simulink model "cloop_AW_1"  (Simulink 7.8)
settings: Solver=FixedStepDiscrete  StartTime=0.0  StopTime=20  FixedStep=ts  RelTol=1e-3
values from neighbouring files (symbols this model uses):
  D_aw = value(U)\value(X)    [AW_synthesis_LMI.m]    (also in Degenerator_test.m = [0 0 0 0])
  satValue = 3.6    [AW_synthesis_LMI.m]    (also in Degenerator_test.m)
  setPoint = 0.015    [Degenerator_test.m]
  ts = 0.005    [identificazione_freq.m]
undefined symbols (not defined in the file or in its folder): N2signal, satSafe
libraries: cstblocks x1
settings Model: Creator=albertoforner  LastModifiedBy=giamm  SimulationMode=external  ExtModeTrigDuration=100000  ExtModeWriteAllDataToWs=on
settings DataIOCC: LimitDataPoints=off
settings DebuggingCC: FrameProcessingCompatibilityMsg=error  StrictBusMsg=Warning
settings HardwareCC: ProdBitPerPointer=64  ProdLargestAtomicFloat=Float  ProdIntDivRoundTo=Zero  ProdEndianess=LittleEndian  ProdHWDeviceType=Specified
settings RTWCC: SystemTargetFile=rtwin.tlc  TemplateMakefile=rtwin.tmf  Description=Simulink Desktop Real-Time  RTWCompilerOptimization=On
settings CodeAppCC: MaxIdLength=95  CustomSymbolStrType=$N$R$M_T
settings RTWinTargetCC: TargetPreCompLibLocation=C:\Program Files\MATLAB\R2016b\toolbox\sldrt\lib\win64  TargetFunctionLibrary=C89/C90 (ANSI)  GeneratePreprocessorConditionals=Use local settings  UseToolchainInfoCompliant=off  ExtModeMexFile=sldrtext

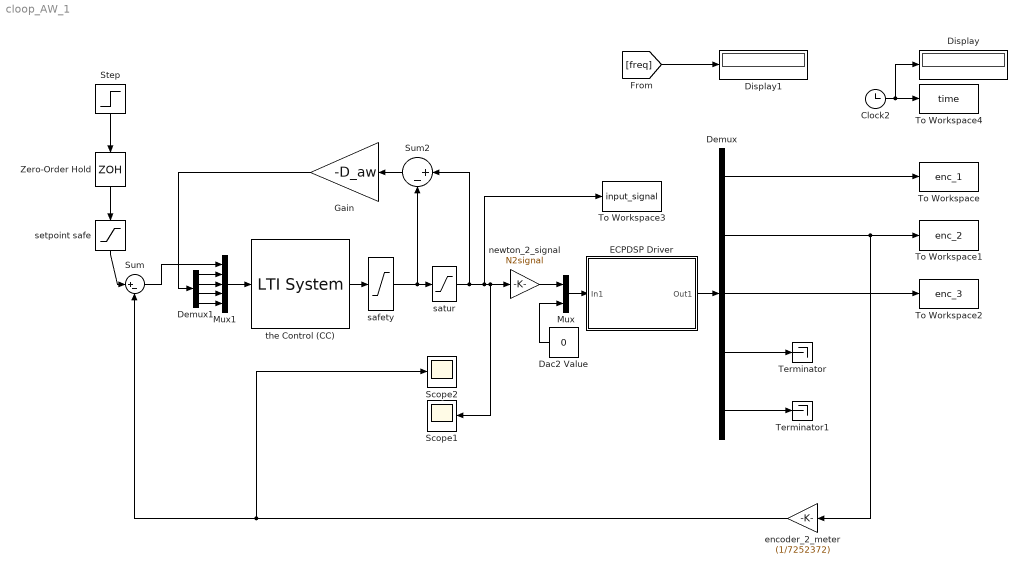
== system cloop_AW_1 ==
  Clock2 : Clock
      settings: DisableCoverage=on
  Dac2 Value : Constant  Value=0  SampleTime=ts
  Demux : Demux  Outputs=5
  Demux1 : Demux
  Display : Display
      settings: Decimation=100
  Display1 : Display
      settings: Decimation=100
  ECPDSP Driver : Subsystem  mask{BaseAddr='0xDE00', STime=ts, TimeOutPer=500, HWAccess=on}
      mask prompts: BaseAddr "Base I/O Address"; STime "Sample Time (Sec)"; TimeOutPer "Timeout Period (500 ~ 2000)"; HWAccess "Hardware Access"
      mask Display: color('black');disp('ECPDSP Driver\n upto\n 4 Encs(ADC Channels)\n and 2 Dacs')
  Gain : Gain  Gain=-D_aw
  Mux : Mux  Inputs=2
  Mux1 : Mux  Inputs=5
  Scope1 : Scope
      settings: TimeRange=auto  MaxDataPoints=5000  SaveToWorkspace=off  YMin=3.5625  YMax=3.9375  SampleTime=-1
  Scope2 : Scope
      settings: TimeRange=auto  MaxDataPoints=5000  SaveToWorkspace=off  SaveName=ScopeData  YMin=-0.03  YMax=0.0275  SampleTime=-1
  Step : Step  Time=ts  After=setPoint  SampleTime=ts
  Sum : Sum  Inputs=|+-
  Sum2 : Sum  Inputs=|+-
  Terminator : Terminator
  Terminator1 : Terminator
  To Workspace : ToWorkspace  VariableName=enc_1  SampleTime=-1
  To Workspace1 : ToWorkspace  VariableName=enc_2  SampleTime=-1
  To Workspace2 : ToWorkspace  VariableName=enc_3  SampleTime=-1
  To Workspace3 : ToWorkspace  VariableName=input_signal  SampleTime=ts
  To Workspace4 : ToWorkspace  VariableName=time  SampleTime=-1
  Zero-Order Hold : ZeroOrderHold  SampleTime=ts
  encoder_2_meter : Gain  Gain=(1/7252372)
  newton_2_signal : Gain  Gain=N2signal
  safety : Saturate  UpperLimit=satSafe  LowerLimit=-satSafe
  satur : Saturate  UpperLimit=satValue  LowerLimit=-satValue
  setpoint safe : Saturate  UpperLimit=0.02  LowerLimit=-0.02
  the Control (CC) : cstblocks/LTI System  sys=CC_1d  IC=[]
  wires:
  Dac2 Value/1 -> Mux/2
  Mux/1 -> ECPDSP Driver/1(In1)
  ECPDSP Driver/1(Out1) -> Demux/1
  Demux/1 -> To Workspace/1
  Demux/2 -> To Workspace1/1, encoder_2_meter/1
  Demux/3 -> To Workspace2/1
  Clock2/1 -> To Workspace4/1, Display/1
  Demux/4 -> Terminator/1
  Demux/5 -> Terminator1/1
  [freq] -> Display1/1
  Step/1 -> Zero-Order Hold/1
  encoder_2_meter/1 -> Sum/2, Scope2/1
  Zero-Order Hold/1 -> setpoint safe/1
  setpoint safe/1 -> Sum/1
  the Control (CC)/1 -> safety/1
  safety/1 -> Sum2/2, satur/1
  newton_2_signal/1 -> Mux/1
  satur/1 -> Sum2/1, To Workspace3/1, newton_2_signal/1, Scope1/1
  Sum2/1 -> Gain/1
  Mux1/1 -> the Control (CC)/1
  Gain/1 -> Demux1/1
  Demux1/1 -> Mux1/2
  Demux1/2 -> Mux1/3
  Demux1/3 -> Mux1/4
  Demux1/4 -> Mux1/5
  Sum/1 -> Mux1/1

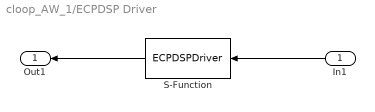
== system cloop_AW_1/ECPDSP Driver ==
  In1 : Inport
  S-Function : S-Function  FunctionName=ECPDSPDriver  Parameters=BaseAddr,STime,TimeOutPer,HWAccess  SFunctionDeploymentMode=off  EnableBusSupport=off
  Out1 : Outport
  wires:
  S-Function/1 -> Out1/1
  In1/1 -> S-Function/1
